simulink model "TercerEjercicio"  (R2021b)
settings: Solver=VariableStepAuto  StartTime=0.0  StopTime=60  RelTol=1e-3
settings Model: Creator=ESTUDIANTE  LastModifiedBy=Brayan
settings SolverCC: AlgebraicLoopSolver=TrustRegion
settings DataIOCC: ReturnWorkspaceOutputs=off
settings DebuggingCC: SFMachineParentedDataDiag=warning  ArithmeticOperatorsInVariantConditions=warning
settings SFSimCC: SimUseLocalCustomCode=off  CustomCodeUndefinedFunction=UseInterfaceOnly
settings RTWCC: RTWUseLocalCustomCode=off

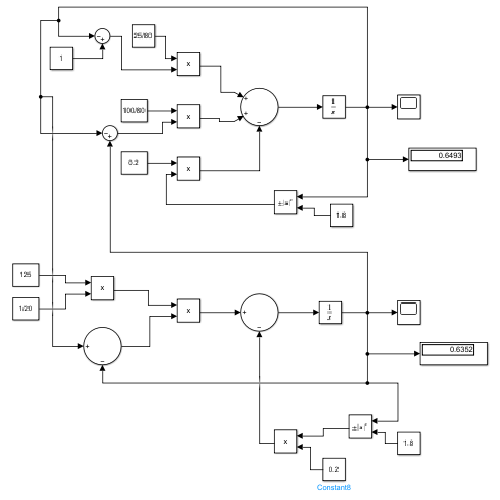
[thumbnail: Simulink's stored preview of the top-level diagram]
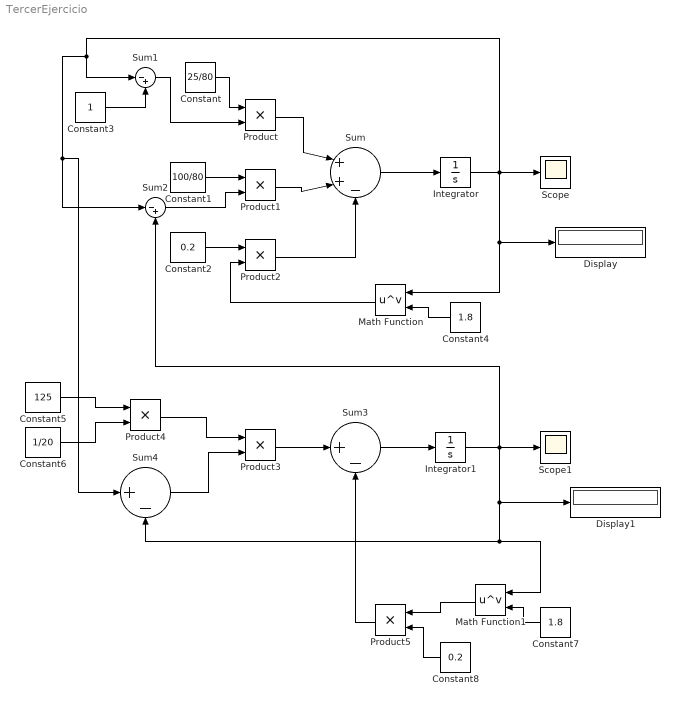
== system TercerEjercicio ==
  Constant : Constant  Value=25/80
  Constant1 : Constant  Value=100/80
  Constant2 : Constant  Value=0.2
  Constant3 : Constant
  Constant4 : Constant  Value=1.8
  Constant5 : Constant  Value=125
  Constant6 : Constant  Value=1/20
  Constant7 : Constant  Value=1.8
  Constant8 : Constant  Value=0.2
  Display : Display
  Display1 : Display
  Integrator : Integrator
  Integrator1 : Integrator
  Math Function : Math  Operator=pow  SignedPower=on  SaturateOnIntegerOverflow=on
  Math Function1 : Math  Operator=pow  SignedPower=on  SaturateOnIntegerOverflow=on
  Product{,1..5} (6 alike) : Product
  Scope : Scope
  Scope1 : Scope
  Sum : Sum  Inputs=|++-
  Sum1 : Sum  Inputs=|-+
  Sum2 : Sum  Inputs=|-+
  Sum3 : Sum  Inputs=|+-
  Sum4 : Sum  Inputs=|+-
  wires:
  Constant/1 -> Product/1
  Product/1 -> Sum/1
  Constant1/1 -> Product1/1
  Product1/1 -> Sum/2
  Constant2/1 -> Product2/1
  Product2/1 -> Sum/3
  Sum/1 -> Integrator/1
  Integrator/1 -> Display/1, Math Function/1, Sum4/1, Sum2/1, Sum1/1, Scope/1
  Sum1/1 -> Product/2
  Constant3/1 -> Sum1/2
  Sum2/1 -> Product1/2
  Math Function/1 -> Product2/2
  Constant4/1 -> Math Function/2
  Sum3/1 -> Integrator1/1
  Integrator1/1 -> Display1/1, Math Function1/1, Sum4/2, Sum2/2, Scope1/1
  Product3/1 -> Sum3/1
  Product4/1 -> Product3/1
  Constant5/1 -> Product4/1
  Constant6/1 -> Product4/2
  Sum4/1 -> Product3/2
  Constant7/1 -> Math Function1/2
  Product5/1 -> Sum3/2
  Math Function1/1 -> Product5/1
  Constant8/1 -> Product5/2
